simulink model "Q_1_6"  (R2018b)
settings: Solver=VariableStepAuto  StartTime=0.0  StopTime=10.0  RelTol=1e-3
libraries: vrlib x1
settings Model: Creator=ASUS  LastModifiedBy=ASUS

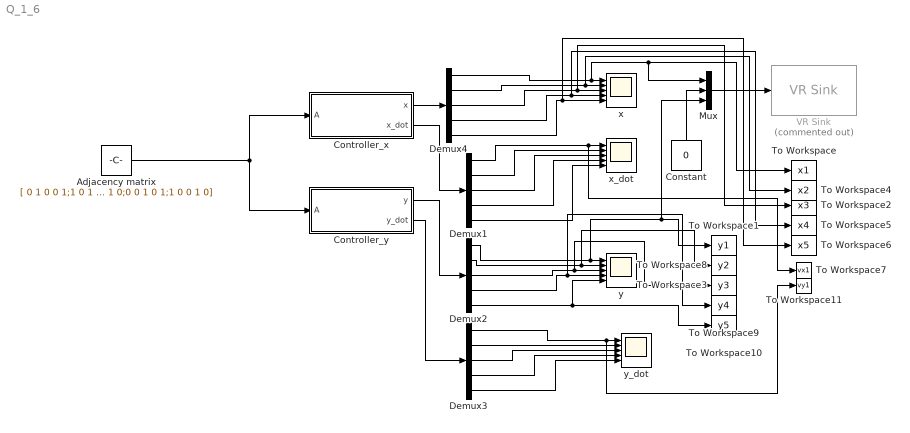
== system Q_1_6 ==
  Adjacency matrix : Constant  Value=[ 0 1 0 0 1;1 0 1 0 0;0 1 0 1 0;0 0 1 0 1;1 0 0 1 0]
  Constant : Constant  Value=0
  Controller_x : Subsystem
  Controller_y : Subsystem
  Demux{1..4} (4 alike) : Demux  Outputs=5
  Mux : Mux  Inputs=3
  To Workspace : ToWorkspace  VariableName=x1  SampleTime=-1
  To Workspace1 : ToWorkspace  VariableName=y1  SampleTime=-1
  To Workspace10 : ToWorkspace  VariableName=y5  SampleTime=-1
  To Workspace11 : ToWorkspace  VariableName=vy1  SampleTime=-1
  To Workspace2 : ToWorkspace  VariableName=x3  SampleTime=-1
  To Workspace3 : ToWorkspace  VariableName=y3  SampleTime=-1
  To Workspace4 : ToWorkspace  VariableName=x2  SampleTime=-1
  To Workspace5 : ToWorkspace  VariableName=x4  SampleTime=-1
  To Workspace6 : ToWorkspace  VariableName=x5  SampleTime=-1
  To Workspace7 : ToWorkspace  VariableName=vx1  SampleTime=-1
  To Workspace8 : ToWorkspace  VariableName=y2  SampleTime=-1
  To Workspace9 : ToWorkspace  VariableName=y4  SampleTime=-1
  VR Sink : vrlib/VR Sink  Commented=on  InstantiateOnLoad=on  SampleTime=0.1  ViewEnable=on  RemoteChange=off  RemoteView=off  FieldsWritten=base.translation.3.1.1.double  WorldFileName=Car1.WRL  AutoView=off  VideoDimensions=[]  AllowVariableSize=off
      settings: SourceProductBaseCode=VR
  x : Scope  NumInputPorts=5
  x_dot : Scope  NumInputPorts=5
  y : Scope  NumInputPorts=5
  y_dot : Scope  NumInputPorts=5
  wires:
  Demux3/4 -> y_dot/4
  Demux3/3 -> y_dot/3
  Demux3/1 -> To Workspace11/1, y_dot/1
  Demux1/4 -> x_dot/4
  Demux2/4 -> y/4, To Workspace9/1
  Demux2/2 -> To Workspace8/1, y/2
  Demux2/3 -> To Workspace3/1, y/3
  Demux1/5 -> x_dot/5
  Controller_x/2(x_dot) -> Demux1/1
  Demux4/4 -> x/4, To Workspace5/1
  Mux/1 -> VR Sink/1
  Demux4/1 -> Mux/1, To Workspace/1, x/1
  Demux4/5 -> x/5, To Workspace6/1
  Demux1/2 -> x_dot/2
  Demux1/1 -> To Workspace7/1, x_dot/1
  Demux2/5 -> To Workspace10/1, y/5
  Controller_y/2(y_dot) -> Demux3/1
  Demux3/5 -> y_dot/5
  Constant/1 -> Mux/2
  Controller_x/1(x) -> Demux4/1
  Demux4/3 -> To Workspace2/1, x/3
  Demux4/2 -> To Workspace4/1, x/2
  Demux3/2 -> y_dot/2
  Demux2/1 -> To Workspace1/1, Mux/3, y/1
  Adjacency matrix/1 -> Controller_x/1(A), Controller_y/1(A)
  Demux1/3 -> x_dot/3
  Controller_y/1("y ") -> Demux2/1

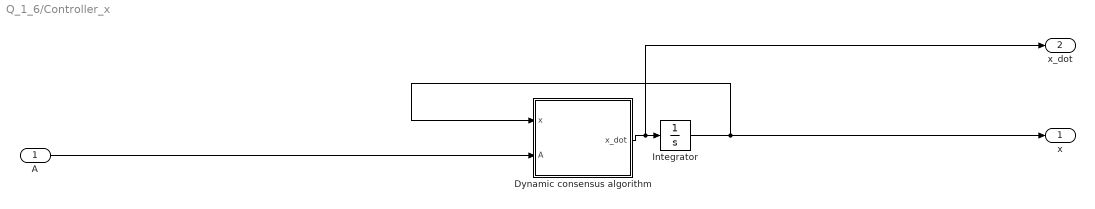
== system Q_1_6/Controller_x ==
  A : Inport
  Dynamic consensus algorithm : MATLAB Function  TreatAsAtomicUnit=on
  Integrator : Integrator  InitialCondition=[-1;3;2;-4;6]
  x : Outport
  x_dot : Outport  Port=2
  wires:
  Integrator/1 -> x/1, Dynamic consensus algorithm/1(x)
  Dynamic consensus algorithm/1(x_dot) -> x_dot/1, Integrator/1
  A/1 -> Dynamic consensus algorithm/2(A)

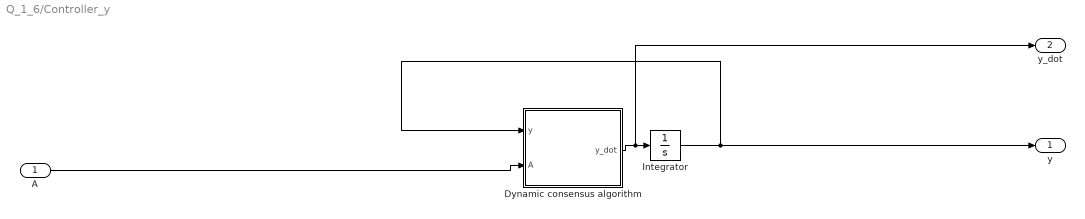
== system Q_1_6/Controller_y ==
  A : Inport
  Dynamic consensus algorithm : MATLAB Function  TreatAsAtomicUnit=on
  Integrator : Integrator  InitialCondition=[4;3;-6;-2;8]
  "y " : Outport
  y_dot : Outport  Port=2
  wires:
  Integrator/1 -> "y "/1, Dynamic consensus algorithm/1(y)
  Dynamic consensus algorithm/1(y_dot) -> y_dot/1, Integrator/1
  A/1 -> Dynamic consensus algorithm/2(A)

== matlab function Q_1_6/Controller_x/Dynamic consensus algorithm ==
  data: x input; x_dot output; A input
function x_dot = con(x,A)
rowsums = sum(A');
[n,n] = size(A);
D = eye(n);
for i = 1:n
   D(i,i) = rowsums(i); 
end
L = D - A;
x_dot = -L*x;

== matlab function Q_1_6/Controller_y/Dynamic consensus algorithm ==
  data: y input; y_dot output; A input
function y_dot = con(y,A)
rowsums = sum(A');
[n,n] = size(A);
D = eye(n);
for i = 1:n
   D(i,i) = rowsums(i); 
end
L = D - A;
y_dot = -L*y;
